simulink model "modelo_planta_EXPERIMENTAL_prueba"  (R2025b)
settings: Solver=FixedStepAuto  StartTime=0.0  StopTime=inf  FixedStep=Ts2  MaxStep=1e-3  RelTol=1e-3
undefined symbols (not defined in the file): ah_max, at_max, bcx, bcy, bh_eq, bhb, bhEb, bhwu, bt, bt_eq, btb, btw, counter_limit, DiscIntNeverNeededParam, g, h_vec_inicial, Hc, ih, is_scanned_vec_inicial, it, Jh_eq, Jt_eq, Kcy, khwu, Ki_h, Ki_t, Kp_h, Kp_t, Ktw, lambda, Lh, Lh0, lh_0, Lt, magnitude, Mc_max, Ms, Mt, N_xt, P_nom, periodo_pulsos, rhd, rtd, tau_hm, tau_tm, Thb_Max, ThEb_Max, Thm_0, Thm_Max, titahm_0, titatm_0, Ts0, Ts1, Ts2, Ttb_Max, Ttm_0, Ttm_Max, vh_0, vh_max_unloaded, vh_nom ... (+20)
libraries: simulink x17, simulink_extras x2, sl3dlib x1, dspnetwork x1
(part 1 of 2)
settings Model: PacingRate=5  Creator=Nahuel  LastModifiedBy=rodri
settings SolverCC: ZeroCrossControl=DisableAll
settings DebuggingCC: UnderSpecifiedDimensionMsg=warning
settings SFSimCC: SimTargetLang=C++  SimDLTargetLibrary=mkl-dnn
settings RTWCC: GPUComputeCapability=3.5
settings ConfigComp: PLC_TargetIDE=codesys35  PLC_MultiTBSigbuilderTimeRange=off  PLC_FoldFBCallOutputVar=off  PLC_RemoveUnusedSSMethodCallArguments=off  PLC_UseCallOutputArgSyntax=off  PLC_EnableUnsignedAndDoubleTypes=off  PLC_EnableUDTSplitting=off  PLC_MaxFieldsInUDT=500.0  PLC_InlineEnumCastFunction=off  PLC_RTWMaxIdLength=31.0  PLC_RollThreshold=5.0  PLC_ActiveTab=0.0  PLC_EnableStringLiteralTB=on  PLC_Enable64bitIntSupport=off

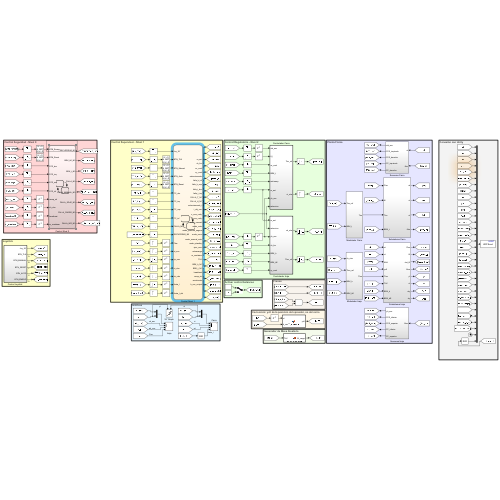
[thumbnail: Simulink's stored preview of the top-level diagram]
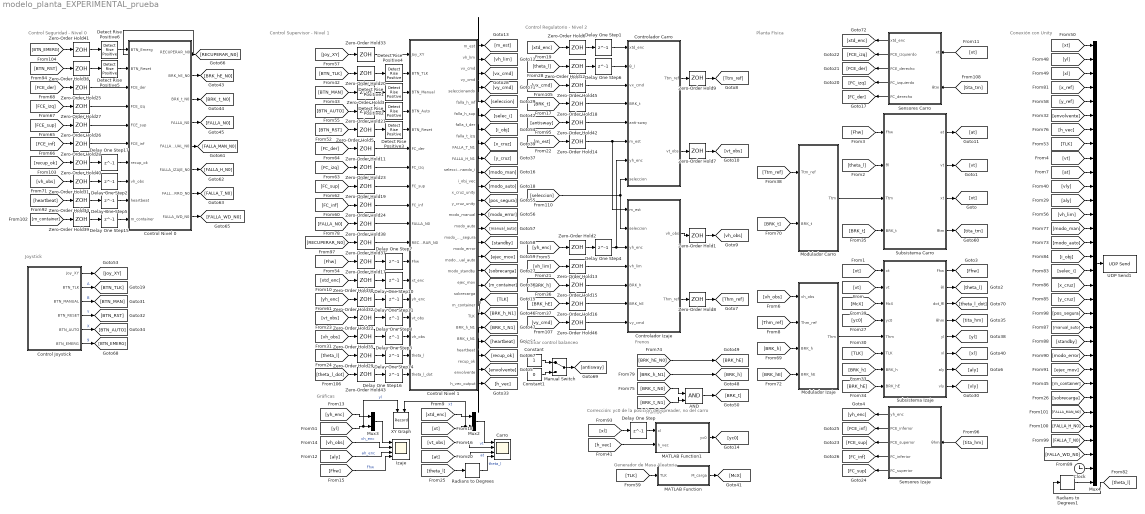
== system modelo_planta_EXPERIMENTAL_prueba ==
  note: Activar control balanceo
  note: Generador de Masa Aleatoria
  note: Frenos
  note: Corrección: yc0 de la posición del spreader, no del carro
  note: Joystick
  note: Control Seguridad - Nivel 0
  note: Control Regulatorio - Nivel 2
  note: Control Supervisor - Nivel 1
  note: Conexión con Unity
  note: Planta Física
  note: Gráficas
  AND : Logic  IconShape=distinctive  AllPortsSameDT=off  OutDataTypeStr=boolean
  Carro : Scope  NumInputPorts=4
      settings: AxesScalingNumUpdates=5  ActiveDisplayYMinimum=-26.90845  ActiveDisplayYMaximum=42.17601
  Clock : Clock
  Constant : Constant
  Constant1 : Constant  Value=0
  "Control Joystick " : Subsystem  TreatAsAtomicUnit=on  SystemSampleTime=Ts2
  Control Nivel 0 : Stateflow chart  Priority=1  TreatAsAtomicUnit=on  SystemSampleTime=Ts0
      settings: PortSchema="{\"entries\":[{\"content\":{\"sides\":[{\"content\":{\"connectorIds\":[\"In1\",\"In7\",\"In2\",\"In5\",\"In3\",\"In6\",\"In10\",\"In4\",\"In8\",\"In9\"]},\"type\":\"ConnectorPlacement.EquallySpacedRectSide\",\"uuid\":\"72248b79-25cb-4c81-9f00-8922a9a1cf34\"},{\"content\":{\"connectorIds\":[\"Out4\",\"Out2\",\"Out3\",\"Out1\",\"Out5\",\"Out6\",\"Out7\",\"Out8\"],\"side\":\"RIGHT\"},\"type\":\"ConnectorPlacement.EquallySpacedRectSide\",\"uuid\":\"f4bfcd12-c204-46a9-9a4b-20ccb9bfcfbb\"},{\"content\":{\"side\":\"TOP\"},\"type\":\"ConnectorPlacement.EquallySpacedRectSide\",\"uuid\":\"f84291a0-0f0e-4f0d-b220-c2febce5b448\"}]},\"type\":\"ConnectorPlacement.EquallySpacedConnector\",\"uuid\":\"3b165743-ae9e-4544-8961-e71410288a4b\"}],\"packageUris\":[\"http://schema.mathworks.com/mf0/Connector/R2020b\"],\"version\":\"1.0\"}"
  Control Nivel 1 : Stateflow chart  Priority=2  TreatAsAtomicUnit=on  SystemSampleTime=Ts1
      settings: PortSchema="{\"entries\":[{\"content\":{\"sides\":[{\"content\":{\"connectorIds\":[\"In5\",\"In4\",\"In6\",\"In7\",\"In8\",\"In9\",\"In11\",\"In10\",\"In12\",\"In15\",\"In16\",\"In3\",\"In18\",\"In13\",\"In2\",\"In14\",\"In17\",\"In1\"]},\"type\":\"ConnectorPlacement.EquallySpacedRectSide\",\"uuid\":\"72765c9f-68bf-44f3-92f3-3edecb9ca866\"},{\"content\":{\"connectorIds\":[\"Out1\",\"Out2\",\"Out22\",\"Out24\",\"Out25\",\"Out26\",\"Out27\",\"Out28\",\"Out29\",\"Out30\",\"Out31\",\"Out9\",\"Out10\",\"Out11\",\"Out12\",\"Out7\",\"Out8\",\"Out13\",\"Out14\",\"Out15\",\"Out16\",\"Out17\",\"Out18\",\"Out19\",\"Out5\",\"Out3\",\"Out4\",\"Out20\",\"Out21\",\"Out23\",\"Out6\"],\"side\":\"RIGHT\"},\"type\":\"ConnectorPlacement.EquallySpacedRectSide\",\"uuid\":\"a6939ff5-eef8-44e2-80ea-5356e254e9e8\"},{\"content\":{\"side\":\"TOP\"},\"type\":\"ConnectorPlacement.EquallySpacedRectSide\",\"uuid\":\"0bd5f797-ecd4-419a-b4ec-9e10260d270a\"},{\"content\":{\"side\":\"BOTTOM\"},\"type\":\"ConnectorPlacement.EquallySpacedRectSide\",\"uuid\":\"7945275f-dab8-4c32-b5c3-f64b82fddda0\"}]},\"type\":\"ConnectorPlacement.EquallySpacedConnector\",\"uuid\":\"3d3cbadb-c70b-461a-afd4-e8d4b160ddcd\"}],\"packageUris\":[\"http://schema.mathworks.com/mf0/Connector/R2020b\"],\"version\":\"1.0\"}"
  Controlador Carro : Subsystem  Priority=3  TreatAsAtomicUnit=on  SystemSampleTime=Ts2
  Controlador Izaje : Subsystem  Priority=3  TreatAsAtomicUnit=on  SystemSampleTime=Ts2
  Delay One Step : Delay  DelayLength=1  InitialCondition=xl_0
  Delay One Step1 : Delay  DelayLength=1  InitialCondition=xtd_0
  Delay One Step10 : Delay  DelayLength=1  InitialCondition=xt_0
  Delay One Step11 : Delay  DelayLength=1  InitialCondition=yh_0
  Delay One Step{2..3,5..6,8,14..17} (9 alike) : Delay  DelayLength=1  InitialCondition=0
  Delay One Step4 : Delay  DelayLength=1  InitialCondition=yh_0
  Delay One Step7 : Delay  DelayLength=1
  Detect Rise Positive{1..6} (6 alike) : simulink/Logic and Bit Operations/Detect Rise Positive  vinit=0  OutDataTypeStr=boolean
  Izaje : Scope  NumInputPorts=4
      settings: ActiveDisplayYMinimum=-22.31965  ActiveDisplayYMaximum=45.47272
  MATLAB Function : MATLAB Function  TreatAsAtomicUnit=on
  MATLAB Function1 : MATLAB Function  TreatAsAtomicUnit=on
  Manual Switch : ManualSwitch
  Modulador Carro : Subsystem
  Modulador Izaje : Subsystem
  Mux2 : Mux  Inputs=2
  Mux3 : Mux  Inputs=2
  Mux4 : Mux  Inputs=32
  Radians to Degrees : simulink_extras/Transformations/Radians to Degrees
  Radians to Degrees1 : simulink_extras/Transformations/Radians to Degrees
  Sensores Carro : Subsystem
  Sensores Izaje : Subsystem
  Subsistema Carro : Subsystem
  Subsistema Izaje : Subsystem
  UDP Send1 : dspnetwork/UDP Send  remoteURL='127.0.0.1'  remotePort=1234  localURL='0.0.0.0'  localPortSource=Automatically determine  localPort=-1  sendBufferSize=8192  sampletime=-1  blockPlatform=HOST  separateLengthPort=0
  XY Graph : Record  NumPorts=2.0  FileSettingsInternal="{\"entries\":[{\"content\":{\"excelSettings\":{\"content\":{},\"type\":\"Streamout.ExcelSettings\"},\"parquetSettings\":{\"content\":{},\"type\":\"Streamout.ParquetSettings\"}},\"type\":\"Streamout.FileSettingStorage\",\"uuid\":\"\"}],\"packageUris\":[\"http:\\/\\/schema.mathworks.com\\/mf0\\/streamout_blocks\\/R2020a\"],\"version\":\"1.0\"}"  FrameSettings=[0, 0]  Layout=[1 1]  SignalsInternal="{\"entries\":[{\"content\":{\"signals\":[{\"content\":{\"blockPath\":[],\"dimensions\":[1],\"domain\":\"\",\"lineColor\":\"#a2142f\",\"plots\":[ 1 ],\"port\":1,\"sid\":[\"\"],\"signalID\":1,\"signalName\":\"yl\"},\"type\":\"RecordBlkView.Signal\",\"uuid\":\"\"},{\"content\":{\"blockPath\":[],\"dimensions\":[1],\"domain\":\"\",\"lineColor\":\"#139fff\",\"plots\":[ 1 ],\"port\":2,\"sid\":[\"\"],\"signalID\":2,\"signalName\":\"xt\"},\"type\":\"RecordBlkView.Signal\",\"uuid\":\"\"}]},\"type\":\"RecordBlkView.InputSignals\",\"uuid\":\"\"}],\"packageUris\":[\"http:\\/\\/schema.mathworks.com\\/mf0\\/streamout_blocks\\/R2020a\"],\"version\":\"1.0\"}"  VisualizationBindings="{\"xyplotplugin\":{\"info\":[{\"series\":[{\"bindingParametersList\":[{\"parameter\":\"X-Axis\",\"signalID\":2,\"signalName\":\"xt\"},{\"parameter\":\"Y-Axis\",\"signalID\":1,\"signalName\":\"yl\"}],\"seriesID\":0}],\"subplotID\":1}]}}"  CompatibilityTag=XY
  Zero-Order Hold{1..2,6..9,12..16,18,42,45..46} (15 alike) : ZeroOrderHold  SampleTime=Ts2
  Zero-Order Hold{3,5,11,17,19..24,29..30,32..33,35,37..38,43} (18 alike) : ZeroOrderHold  SampleTime=Ts1
  Zero-Order Hold{25..28,31,34,36,39..41} (10 alike) : ZeroOrderHold  SampleTime=Ts0
  wires:
  [Thm_ref] -> Modulador Izaje/2(Thm_ref)
  [vh_obs] -> Izaje/2  "vh_enc"
  Sensores Izaje/4(FC_inferior) -> [FC_inf]
  Delay One Step4/1 -> Controlador Carro/7(yh_enc), Controlador Izaje/3(yh_enc)
  Sensores Izaje/1(yh_enc) -> [yh_enc]
  [BRK_hE] -> Subsistema Izaje/8(BRK_hE)
  Subsistema Izaje/1(Fhw) -> [Fhw]
  Controlador Izaje/2(Thm_ref) -> Zero-Order Hold8/1
  [xt] -> Sensores Carro/1(xt)
  [BRK_h] -> Subsistema Izaje/7(BRK_h)
  Sensores Carro/4(FC_izquierdo) -> [FC_izq]
  [m_est] -> Zero-Order Hold14/1
  Zero-Order Hold2/1 -> Delay One Step4/1
  Zero-Order Hold6/1 -> Delay One Step1/1
  Subsistema Carro/1(at) -> [at]
  [theta_l] -> Subsistema Carro/2(θl)
  [vt] -> Subsistema Izaje/2(vt)
  [xt] -> Subsistema Izaje/1(xt)
  Delay One Step1/1 -> Controlador Carro/1(xtd_enc)
  [aly] -> Izaje/3  "ah_enc"
  Zero-Order Hold8/1 -> [Thm_ref]
  [vh_lim] -> Zero-Order Hold13/1
  Subsistema Carro/3(xt) -> [xt]
  [Fhw] -> Subsistema Carro/1(Fhw)
  Sensores Carro/2(FCE_izquierdo) -> [FCE_izq]
  [yh_enc] -> Zero-Order Hold2/1
  [xtd_enc] -> Zero-Order Hold6/1
  Zero-Order Hold9/1 -> [Ttm_ref]
  Controlador Carro/1(Ttm_ref) -> Zero-Order Hold9/1
  [TLK] -> Subsistema Izaje/6(TLK)
  Sensores Izaje/2(FCE_inferior) -> [FCE_inf]
  Sensores Izaje/3(FCE_superior) -> [FCE_sup]
  Sensores Izaje/5(FC_superior) -> [FC_sup]
  Sensores Carro/3(FCE_derecho) -> [FCE_der]
  Subsistema Izaje/2(θl) -> [theta_l]
  [McX] -> Subsistema Izaje/3(McX)
  Subsistema Carro/2(vt) -> [vt]
  Sensores Carro/5(FC_derecho) -> [FC_der]
  [BRK_t] -> Subsistema Carro/4(BRK_t)
  [BRK_h] -> Zero-Order Hold15/1
  [BRK_hE] -> Zero-Order Hold16/1
  [Ttm_ref] -> Modulador Carro/1(Ttm_ref)
  [BRK_t] -> Zero-Order Hold18/1
  [yh_enc] -> Mux3/1
  [vh_obs] -> Modulador Izaje/1(vh_obs)
  Delay One Step6/1 -> Controlador Carro/2(θ_l)
  [theta_l] -> Zero-Order Hold12/1
  Zero-Order Hold12/1 -> Delay One Step6/1
  Modulador Izaje/1(Thm) -> Subsistema Izaje/5(Thm)
  Modulador Carro/1(Ttm) -> Subsistema Carro/3(Ttm)
  Mux3/1 -> Izaje/1
  Subsistema Izaje/5(yl) -> [yl]
  Subsistema Izaje/6(xl) -> [xl]
  [Fhw] -> Izaje/4  "Fhw"
  Subsistema Izaje/7(aly) -> [aly]
  [yl] -> Mux3/2, XY Graph/1  "yl"
  Control Nivel 1/1(m_est) -> [m_est]
  Control Nivel 1/2(vh_lim) -> [vh_lim]
  Zero-Order Hold13/1 -> Controlador Izaje/4(vh_lim)
  Zero-Order Hold14/1 -> Controlador Izaje/1(m_est), Controlador Carro/6(m_est)
  Zero-Order Hold15/1 -> Controlador Izaje/5(BRK_h)
  Zero-Order Hold16/1 -> Controlador Izaje/6(BRK_hE)
  Zero-Order Hold17/1 -> Delay One Step7/1
  Delay One Step7/1 -> Control Nivel 1/3(Fhw)
  [Fhw] -> Zero-Order Hold17/1
  Zero-Order Hold18/1 -> Controlador Carro/4(BRK_t)
  [BTN_TLK] -> Zero-Order Hold20/1
  Zero-Order Hold20/1 -> Detect Rise Positive4/1
  Zero-Order Hold11/1 -> Control Nivel 1/9(FC_der)
  Zero-Order Hold19/1 -> Control Nivel 1/10(FC_sup)
  Zero-Order Hold23/1 -> Control Nivel 1/11(FC_izq)
  Zero-Order Hold24/1 -> Control Nivel 1/12(FC_inf)
  [FC_izq] -> Zero-Order Hold23/1
  [FC_der] -> Zero-Order Hold11/1
  [FC_sup] -> Zero-Order Hold19/1
  [FC_inf] -> Zero-Order Hold24/1
  Zero-Order Hold25/1 -> Control Nivel 0/2(FCE_der)
  Zero-Order Hold26/1 -> Control Nivel 0/3(FCE_sup)
  Zero-Order Hold27/1 -> Control Nivel 0/5(FCE_izq)
  Zero-Order Hold28/1 -> Control Nivel 0/6(FCE_inf)
  [FCE_der] -> Zero-Order Hold25/1
  [FCE_izq] -> Zero-Order Hold27/1
  [FCE_sup] -> Zero-Order Hold26/1
  [FCE_inf] -> Zero-Order Hold28/1
  [BRK_h] -> Modulador Izaje/3(BRK_h)
  [vh_obs] -> Zero-Order Hold31/1
  Zero-Order Hold31/1 -> Delay One Step2/1
  [BRK_hE] -> Modulador Izaje/4(BRK_hE)
  [BRK_t] -> Modulador Carro/2(BRK_t)
  Control Nivel 0/2(BRK_hE_N0) -> [BRK_hE_N0]
  Control Nivel 0/3(BRK_t_N0) -> [BRK_t_N0]
  [xtd_enc] -> Zero-Order Hold30/1
  [yh_enc] -> Zero-Order Hold32/1
  Zero-Order Hold30/1 -> Delay One Step10/1
  Zero-Order Hold32/1 -> Delay One Step11/1
  Delay One Step11/1 -> Control Nivel 1/13(yh_enc)
  Control Nivel 0/1(FALLA_N0) -> [FALLA_N0]
  [FALLA_N0] -> Zero-Order Hold38/1
  Control Nivel 1/3(BRK_h_N1) -> [BRK_h_N1]
  Control Nivel 1/4(BRK_t_N1) -> [BRK_t_N1]
  [BRK_t_N0] -> AND/1
  [BRK_t_N1] -> AND/2
  [BRK_h_N1] -> [BRK_h]
  [BRK_hE_N0] -> [BRK_hE]
  AND/1 -> [BRK_t]
  [BTN_MAN] -> Zero-Order Hold3/1
  Zero-Order Hold38/1 -> Control Nivel 1/15(FALLA_N0)
  "Control Joystick "/2(BTN_TLK) -> [BTN_TLK]  "A"
  "Control Joystick "/1(Joy_XY) -> [Joy_XY]
  [Joy_XY] -> Zero-Order Hold33/1
  Zero-Order Hold33/1 -> Control Nivel 1/5(Joy_XY)
  Control Nivel 1/5(TLK) -> [TLK]
  Delay One Step16/1 -> Control Nivel 1/1(theta_l_dot)
  Control Nivel 1/6(h_vec_output) -> [h_vec]
  Subsistema Izaje/8(vly) -> [vly]
  "Control Joystick "/5(BTN_AUTO) -> [BTN_AUTO]  "X"
  "Control Joystick "/4(BTN_RESET) -> [BTN_RST]  "Y"
  "Control Joystick "/3(BTN_MANUAL) -> [BTN_MAN]  "B"
  Zero-Order Hold3/1 -> Detect Rise Positive1/1
  [BTN_AUTO] -> Zero-Order Hold21/1
  Zero-Order Hold21/1 -> Detect Rise Positive2/1
  [BTN_RST] -> Zero-Order Hold5/1
  Zero-Order Hold5/1 -> Detect Rise Positive3/1
  [TLK] -> MATLAB Function/1(TLK)
  MATLAB Function/1(M_carga) -> [McX]
  [vh_lim] -> Mux4/13
  [at] -> Mux4/10
  [vt] -> Mux4/9
  [xt] -> Mux4/1
  [envolvente] -> Mux4/6
  [vly] -> Mux4/11
  [h_vec] -> Mux4/7
  [yl] -> Mux4/2
  [y_ref] -> Mux4/5
  [TLK] -> Mux4/8
  [xl] -> Mux4/3
  [x_ref] -> Mux4/4
  Mux4/1 -> UDP Send1/1
  [vt_obs] -> Zero-Order Hold22/1
  Zero-Order Hold22/1 -> Delay One Step8/1
  Delay One Step8/1 -> Control Nivel 1/2(vt_obs)
  [theta_l] -> Zero-Order Hold29/1
  Zero-Order Hold29/1 -> Delay One Step14/1
  Delay One Step14/1 -> Control Nivel 1/17(theta_l)
  Control Nivel 1/7(modo_manual) -> [modo_man]
  Control Nivel 1/8(modo_auto) -> [modo_auto]
  [modo_man] -> Mux4/14
  [modo_auto] -> Mux4/15
  Control Nivel 1/12(y_cruz_unity) -> [y_cruz]
  Control Nivel 1/11(x_cruz_unity) -> [x_cruz]
  Control Nivel 1/9(seleccionando_i) -> [selec_i]
  Control Nivel 1/10(i_obj_vec) -> [i_obj]
  [i_obj] -> Mux4/16
  [selec_i] -> Mux4/17
  [x_cruz] -> Mux4/18
  [y_cruz] -> Mux4/19
  Control Nivel 1/13(modo_posicion_segura) -> [pos_segura]
  Control Nivel 1/14(modo_error) -> [modo_error]
  Control Nivel 1/15(modo_manual_auto) -> [manual_auto]
  Control Nivel 1/16(modo_standby) -> [standby]
  [pos_segura] -> Mux4/20
  [manual_auto] -> Mux4/21
  [standby] -> Mux4/22
  [modo_error] -> Mux4/23
  Control Nivel 1/17(ejec_mov) -> [ejec_mov]
  [ejec_mov] -> Mux4/24
  Control Nivel 1/19(m_container) -> [m_container]
  Control Nivel 1/18(sobrecarga) -> [sobrecarga]
  [m_container] -> Mux4/25
  [sobrecarga] -> Mux4/26
  MATLAB Function1/1(yc0) -> [yc0]
  [xl] -> Delay One Step/1
  Delay One Step/1 -> MATLAB Function1/1(xl)
  [h_vec] -> MATLAB Function1/2(h_vec)
  [yc0] -> Subsistema Izaje/4(yc0)
  [BTN_RST] -> Zero-Order Hold36/1
  [aly] -> Mux4/12
  Control Nivel 0/5(FALLA_MANUAL_N0) -> [FALLA_MAN_N0]
  Control Nivel 0/6(FALLA_IZAJE_N0) -> [FALLA_H_N0]
  Control Nivel 0/7(FALLA_CARRO_N0) -> [FALLA_T_N0]
  Control Nivel 1/20(heartbeat) -> [heartbeat]
  [heartbeat] -> Zero-Order Hold34/1
  Zero-Order Hold34/1 -> Delay One Step5/1
  Zero-Order Hold36/1 -> Detect Rise Positive5/1
  Delay One Step5/1 -> Control Nivel 0/8(heartbeat)
  Control Nivel 0/8(FALLA_WD_N0) -> [FALLA_WD_N0]
  [FALLA_MAN_N0] -> Mux4/27
  [FALLA_H_N0] -> Mux4/28
  [FALLA_T_N0] -> Mux4/29
  [FALLA_WD_N0] -> Mux4/30
  Control Nivel 0/4(RECUPERAR_N0) -> [RECUPERAR_N0]
  [RECUPERAR_N0] -> Zero-Order Hold37/1
  Zero-Order Hold37/1 -> Control Nivel 1/16(RECUPERAR_N0)
  [m_container] -> Zero-Order Hold39/1
  Zero-Order Hold39/1 -> Delay One Step15/1
  Delay One Step15/1 -> Control Nivel 0/9(m_container)
  Control Nivel 1/21(recup_ok) -> [recup_ok]
  [recup_ok] -> Zero-Order Hold40/1
  Zero-Order Hold40/1 -> Delay One Step17/1
  "Control Joystick "/6(BTN_EMERG) -> [BTN_EMERG]  "9"
  Zero-Order Hold41/1 -> Detect Rise Positive6/1
  [BTN_EMERG] -> Zero-Order Hold41/1
  Detect Rise Positive1/1 -> Control Nivel 1/6(BTN_Manual)
  Detect Rise Positive2/1 -> Control Nivel 1/7(BTN_Auto)
  Detect Rise Positive3/1 -> Control Nivel 1/8(BTN_Reset)
  Detect Rise Positive4/1 -> Control Nivel 1/4(BTN_TLK)
  Detect Rise Positive5/1 -> Control Nivel 0/7(BTN_Reset)
  Detect Rise Positive6/1 -> Control Nivel 0/1(BTN_Emerg)
  Zero-Order Hold42/1 -> Controlador Carro/5(anti-sway)
  [antisway] -> Zero-Order Hold42/1
  Mux2/1 -> Carro/1
  [theta_l] -> Radians to Degrees/1
  [xt] -> Mux2/2, XY Graph/2  "xt"
  [vt_obs] -> Carro/2  "vt"
  Radians to Degrees/1 -> Carro/4  "theta_l"
  [at] -> Carro/3  "at"
  [xtd_enc] -> Mux2/1
  [theta_l_dot] -> Zero-Order Hold43/1
  Zero-Order Hold43/1 -> Delay One Step16/1
  Subsistema Izaje/3(dot_θl) -> [theta_l_dot]
  Control Nivel 1/22(vx_cmd) -> [vx_cmd]
  Control Nivel 1/24(vy_cmd) -> [vy_cmd]
  [vx_cmd] -> Zero-Order Hold45/1
  Zero-Order Hold45/1 -> Controlador Carro/3(vx_cmd)
  [vy_cmd] -> Zero-Order Hold46/1
  Zero-Order Hold46/1 -> Controlador Izaje/7(vy_cmd)
  Controlador Carro/2(vt_obs) -> Zero-Order Hold7/1
  Zero-Order Hold7/1 -> [vt_obs]
  Delay One Step10/1 -> Control Nivel 1/18(xt_enc)
  Sensores Carro/1(xtd_enc) -> [xtd_enc]
  Controlador Izaje/1(vh_obs) -> Zero-Order Hold1/1
  Zero-Order Hold1/1 -> [vh_obs]
  Delay One Step2/1 -> Control Nivel 0/4(vh_obs)
  Constant/1 -> Manual Switch/1
  Manual Switch/1 -> [antisway]
  Constant1/1 -> Manual Switch/2
  [vh_obs] -> Zero-Order Hold35/1
  Zero-Order Hold35/1 -> Delay One Step3/1
  Delay One Step3/1 -> Control Nivel 1/14(vh_obs)
  Control Nivel 1/23(envolvente) -> [envolvente]
  Delay One Step17/1 -> Control Nivel 0/10(recup_ok)
  Subsistema Izaje/4(θhm) -> [tita_hm]
  [tita_hm] -> Sensores Izaje/1(θhm)
  Subsistema Carro/4(θtm) -> [tita_tm]
  [tita_tm] -> Sensores Carro/2(θtm)
  Clock/1 -> Mux4/31
  [theta_l] -> Radians to Degrees1/1
  Radians to Degrees1/1 -> Mux4/32
  Control Nivel 1/25(seleccionando) -> [seleccion]
  [seleccion] -> Controlador Izaje/2(seleccion), Controlador Carro/8(seleccion)

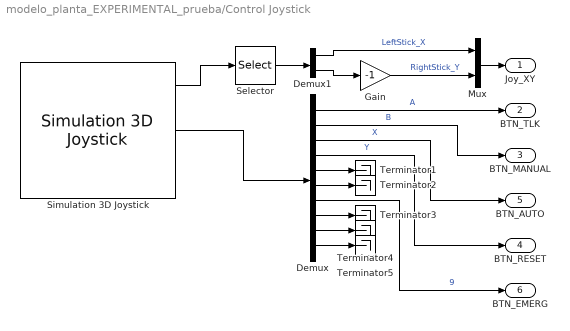
== system modelo_planta_EXPERIMENTAL_prueba/Control Joystick  ==
  Demux : Demux  Outputs=10
  Demux1 : Demux  Outputs=2
  Gain : Gain  Gain=-1
  Mux : Mux  Inputs=2
  Selector : Selector  InputPortWidth=5  IndexOptions=Index vector (dialog)  Indices=[1 5]  OutputSizes=1
  Simulation 3D Joystick : sl3dlib/Simulation 3D/Hardware Interface/Simulation 3D Joystick  joyid=1  adjustports=on  forcefeed=off
  Terminator{1..5} (5 alike) : Terminator
  Joy_XY : Outport
  BTN_TLK : Outport  Port=2
  BTN_MANUAL : Outport  Port=3
  BTN_RESET : Outport  Port=4
  BTN_AUTO : Outport  Port=5
  BTN_EMERG : Outport  Port=6
  wires:
  Demux/1 -> BTN_TLK/1  "A"
  Demux1/2 -> Gain/1
  Demux1/1 -> Mux/1  "LeftStick_X"
  Selector/1 -> Demux1/1
  Simulation 3D Joystick/1 -> Selector/1
  Gain/1 -> Mux/2  "RightStick_Y"
  Simulation 3D Joystick/2 -> Demux/1
  Demux/2 -> BTN_MANUAL/1  "B"
  Demux/3 -> BTN_AUTO/1  "X"
  Demux/4 -> BTN_RESET/1  "Y"
  Mux/1 -> Joy_XY/1
  Demux/5 -> Terminator1/1
  Demux/6 -> Terminator2/1
  Demux/8 -> Terminator3/1
  Demux/9 -> Terminator4/1
  Demux/10 -> Terminator5/1
  Demux/7 -> BTN_EMERG/1  "9"

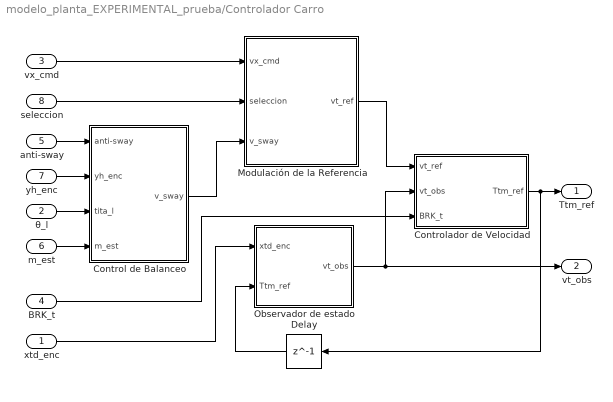
== system modelo_planta_EXPERIMENTAL_prueba/Controlador Carro ==
  xtd_enc : Inport
  θ_l : Inport  Port=2
  vx_cmd : Inport  Port=3
  BRK_t : Inport  Port=4
  anti-sway : Inport  Port=5
  m_est : Inport  Port=6
  yh_enc : Inport  Port=7
  seleccion : Inport  Port=8
  Control de Balanceo : Subsystem
  Controlador de Velocidad : Subsystem
  Delay : Delay  DelayLength=1  InitialCondition=Ttm_0
  Modulación de la Referencia : Subsystem
  Observador de estado : Subsystem  TreatAsAtomicUnit=on  SystemSampleTime=Ts2
  Ttm_ref : Outport
  vt_obs : Outport  Port=2
  wires:
  Modulación de la Referencia/1(vt_ref) -> Controlador de Velocidad/1(vt_ref)
  Controlador de Velocidad/1(Ttm_ref) -> Ttm_ref/1, Delay/1
  xtd_enc/1 -> Observador de estado/1(xtd_enc)
  Delay/1 -> Observador de estado/2(Ttm_ref)
  Control de Balanceo/1(v_sway) -> Modulación de la Referencia/3(v_sway)
  yh_enc/1 -> Control de Balanceo/2(yh_enc)
  θ_l/1 -> Control de Balanceo/3(tita_l)
  m_est/1 -> Control de Balanceo/4(m_est)
  BRK_t/1 -> Controlador de Velocidad/3(BRK_t)
  vx_cmd/1 -> Modulación de la Referencia/1(vx_cmd)
  anti-sway/1 -> Control de Balanceo/1(anti-sway)
  Observador de estado/1(vt_obs) -> Controlador de Velocidad/2(vt_obs), vt_obs/1
  seleccion/1 -> Modulación de la Referencia/2(seleccion)

== system modelo_planta_EXPERIMENTAL_prueba/Controlador Izaje ==
  m_est : Inport
  seleccion : Inport  Port=2
  yh_enc : Inport  Port=3
  vh_lim : Inport  Port=4
  BRK_h : Inport  Port=5
  BRK_hE : Inport  Port=6
  vy_cmd : Inport  Port=7
  AND : Logic  IconShape=distinctive  AllPortsSameDT=off  OutDataTypeStr=boolean
  Controlador de Velocidad : Subsystem  TreatAsAtomicUnit=on  SystemSampleTime=Ts2
  Delay One Step : Delay  DelayLength=1  InitialCondition=Thm_0
  Modulación de la Referencia : Subsystem  TreatAsAtomicUnit=on  SystemSampleTime=Ts2
  Observador de estado : Subsystem  TreatAsAtomicUnit=on  SystemSampleTime=Ts2
  vh_obs : Outport
  Thm_ref : Outport  Port=2
  wires:
  yh_enc/1 -> Observador de estado/1(yh_enc)
  Observador de estado/1(vh_obs) -> Controlador de Velocidad/3(vh_obs), vh_obs/1
  Modulación de la Referencia/1(vh_ref) -> Controlador de Velocidad/2(vh_ref)
  vh_lim/1 -> Modulación de la Referencia/1(vh_lim)
  AND/1 -> Controlador de Velocidad/4(BRK)
  Controlador de Velocidad/1(Thm_ref) -> Delay One Step/1, Thm_ref/1
  Delay One Step/1 -> Observador de estado/2(Thm_ref)
  m_est/1 -> Controlador de Velocidad/1(m_est)
  BRK_h/1 -> AND/1
  BRK_hE/1 -> AND/2
  vy_cmd/1 -> Modulación de la Referencia/3(vy_cmd)
  seleccion/1 -> Modulación de la Referencia/2(seleccion)

== system modelo_planta_EXPERIMENTAL_prueba/Modulador Carro ==
  Ttm_ref : Inport
  BRK_t : Inport  Port=2
  Constant1 : Constant  Value=0
  Gain2 : Gain  Gain=1/tau_tm
  Integrator : Integrator  InitialCondition=Ttm_0
  Saturation : Saturate  UpperLimit=Ttm_Max  LowerLimit=-Ttm_Max
  Sum : Sum  Inputs=|+-
  Switch : Switch  Criteria=u2 > Threshold  SaturateOnIntegerOverflow=off  InputSameDT=off
  Ttm : Outport
  wires:
  Saturation/1 -> Sum/1  "Ttm_lim"
  Sum/1 -> Gain2/1
  Gain2/1 -> Integrator/1
  Integrator/1 -> Ttm/1, Sum/2
  Ttm_ref/1 -> Switch/1
  BRK_t/1 -> Switch/2
  Switch/1 -> Saturation/1
  Constant1/1 -> Switch/3

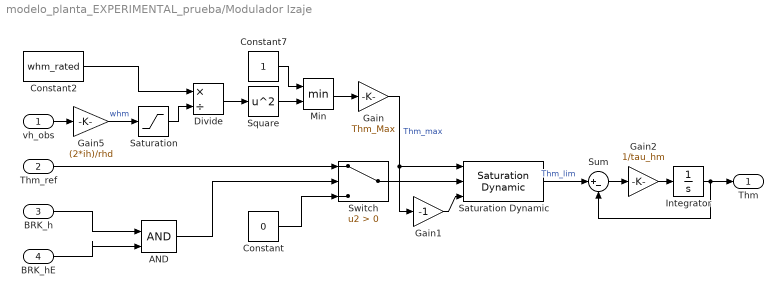
== system modelo_planta_EXPERIMENTAL_prueba/Modulador Izaje ==
  vh_obs : Inport
  Thm_ref : Inport  Port=2
  BRK_h : Inport  Port=3
  BRK_hE : Inport  Port=4
  AND : Logic  IconShape=distinctive  AllPortsSameDT=off  OutDataTypeStr=boolean
  Constant : Constant  Value=0
  Constant2 : Constant  Value=whm_rated
  Constant7 : Constant
  Divide : Product  Inputs=*/
  Gain : Gain  Gain=Thm_Max
  Gain1 : Gain  Gain=-1
  Gain2 : Gain  Gain=1/tau_hm
  Gain5 : Gain  Gain=(2*ih)/rhd
  Integrator : Integrator  InitialCondition=Thm_0
  Min : MinMax  Inputs=2
  Saturation : Saturate  UpperLimit=inf  LowerLimit=whm_rated
  Saturation Dynamic : simulink/Discontinuities/Saturation Dynamic  OutMin=[]  OutMax=[]  OutDataTypeStr=Inherit: Same as second input  OutDataType=fixdt(1, 16)  OutScaling=2^-10  DoSatur=off
  Square : Math  Operator=square
  Sum : Sum  Inputs=|+-
  Switch : Switch  Criteria=u2 > Threshold  SaturateOnIntegerOverflow=off  InputSameDT=off
  Thm : Outport
  wires:
  Constant2/1 -> Divide/1
  Min/1 -> Gain/1
  Constant7/1 -> Min/1
  Gain/1 -> Gain1/1, Saturation Dynamic/1  "Thm_max"
  Saturation/1 -> Divide/2
  Square/1 -> Min/2
  Divide/1 -> Square/1
  vh_obs/1 -> Gain5/1
  Gain1/1 -> Saturation Dynamic/3
  Saturation Dynamic/1 -> Sum/1  "Thm_lim"
  Sum/1 -> Gain2/1
  Gain2/1 -> Integrator/1
  Integrator/1 -> Thm/1, Sum/2
  Thm_ref/1 -> Switch/1
  BRK_h/1 -> AND/1
  Switch/1 -> Saturation Dynamic/2
  BRK_hE/1 -> AND/2
  AND/1 -> Switch/2
  Gain5/1 -> Saturation/1  "whm"
  Constant/1 -> Switch/3

== system modelo_planta_EXPERIMENTAL_prueba/Sensores Carro ==
  xt : Inport
  θtm : Inport  Port=2
  Encoder Carro : Subsystem
  Fines de carrera carro (rieles) : Subsystem
  xtd_enc : Outport
  FCE_izquierdo : Outport  Port=2
  FCE_derecho : Outport  Port=3
  FC_izquierdo : Outport  Port=4
  FC_derecho : Outport  Port=5
  wires:
  Fines de carrera carro (rieles)/1(FC_derecho) -> FC_derecho/1
  θtm/1 -> Encoder Carro/1(θtm)
  Fines de carrera carro (rieles)/2(FC_izquierdo) -> FC_izquierdo/1
  Fines de carrera carro (rieles)/3(FCE_derecho) -> FCE_derecho/1
  Fines de carrera carro (rieles)/4(FCE_izquierdo) -> FCE_izquierdo/1
  xt/1 -> Fines de carrera carro (rieles)/1(xt)
  Encoder Carro/1(xtd_enc) -> xtd_enc/1

== system modelo_planta_EXPERIMENTAL_prueba/Sensores Izaje ==
  θhm : Inport
  Encoder Izaje : Subsystem
  Fines de carrera izaje (tambor) : Subsystem
  yh_enc : Outport
  FCE_inferior : Outport  Port=2
  FCE_superior : Outport  Port=3
  FC_inferior : Outport  Port=4
  FC_superior : Outport  Port=5
  wires:
  Fines de carrera izaje (tambor)/1(FC_superior) -> FC_superior/1
  Fines de carrera izaje (tambor)/4(FCE_inferior) -> FCE_inferior/1
  Fines de carrera izaje (tambor)/2(FC_inferior) -> FC_inferior/1
  Encoder Izaje/1(yh_enc) -> Fines de carrera izaje (tambor)/1(y_enc), yh_enc/1
  θhm/1 -> Encoder Izaje/1(θhm)
  Fines de carrera izaje (tambor)/3(FCE_superior) -> FCE_superior/1

== system modelo_planta_EXPERIMENTAL_prueba/Subsistema Carro ==
  Fhw : Inport
  θl : Inport  Port=2
  Ttm : Inport  Port=3
  BRK_t : Inport  Port=4
  Accionamiento carro : Subsystem
  Dinámica carro : Subsystem
  Fuerza cable carro : Subsystem
  at : Outport
  vt : Outport  Port=2
  xt : Outport  Port=3
  θtm : Outport  Port=4
  wires:
  [Ftw] -> Accionamiento carro/1(Ftw)
  Accionamiento carro/1(θtm) -> θtm/1
  Dinámica carro/1(xt) -> Fuerza cable carro/3(xt), xt/1
  BRK_t/1 -> Accionamiento carro/3(BRK_t)
  [Ftw] -> Dinámica carro/1(Ftw)
  θl/1 -> Dinámica carro/2(θl)
  Ttm/1 -> Accionamiento carro/2(Ttm)
  Fuerza cable carro/1(Ftw) -> [Ftw]
  Dinámica carro/2(vt) -> Fuerza cable carro/4(vt), vt/1
  Accionamiento carro/2(xtd) -> Fuerza cable carro/1(xtd)
  Accionamiento carro/3(vtd) -> Fuerza cable carro/2(vtd)
  Fhw/1 -> Dinámica carro/3(Fhw)
  Dinámica carro/3(at) -> at/1

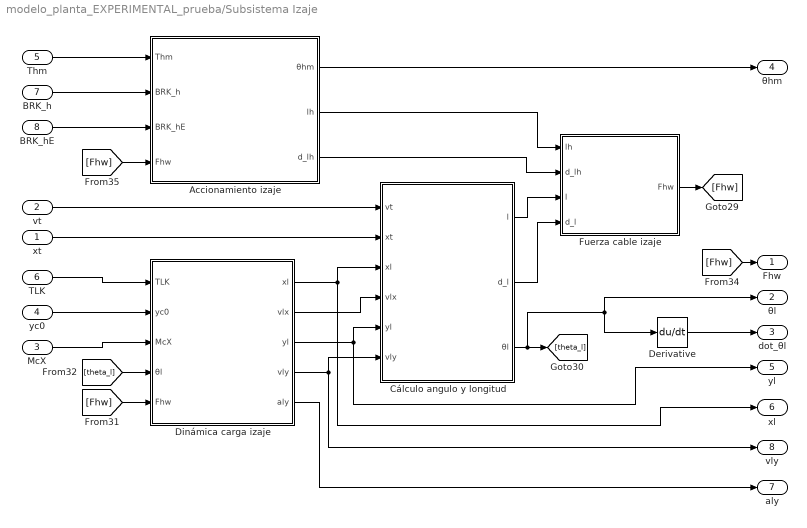
== system modelo_planta_EXPERIMENTAL_prueba/Subsistema Izaje ==
  xt : Inport
  vt : Inport  Port=2
  McX : Inport  Port=3
  yc0 : Inport  Port=4
  Thm : Inport  Port=5
  TLK : Inport  Port=6
  BRK_h : Inport  Port=7
  BRK_hE : Inport  Port=8
  Accionamiento izaje : Subsystem
  Cálculo angulo y longitud : Subsystem
  Derivative : Derivative
  Dinámica carga izaje : Subsystem
  Fuerza cable izaje : Subsystem
  Fhw : Outport
  θl : Outport  Port=2
  dot_θl : Outport  Port=3
  θhm : Outport  Port=4
  yl : Outport  Port=5
  xl : Outport  Port=6
  aly : Outport  Port=7
  vly : Outport  Port=8
  wires:
  vt/1 -> Cálculo angulo y longitud/1(vt)
  Accionamiento izaje/2(lh) -> Fuerza cable izaje/1(lh)
  yc0/1 -> Dinámica carga izaje/2(yc0)
  McX/1 -> Dinámica carga izaje/3(McX)
  Dinámica carga izaje/4(vly) -> vly/1, Cálculo angulo y longitud/6(vly)
  [Fhw] -> Accionamiento izaje/4(Fhw)
  [theta_l] -> Dinámica carga izaje/4(θl)
  xt/1 -> Cálculo angulo y longitud/2(xt)
  BRK_h/1 -> Accionamiento izaje/2(BRK_h)
  Dinámica carga izaje/1(xl) -> Cálculo angulo y longitud/3(xl), xl/1
  Dinámica carga izaje/2(vlx) -> Cálculo angulo y longitud/4(vlx)
  Fuerza cable izaje/1(Fhw) -> [Fhw]
  Cálculo angulo y longitud/1(l) -> Fuerza cable izaje/3(l)
  Accionamiento izaje/1(θhm) -> θhm/1
  Cálculo angulo y longitud/3(θl) -> θl/1, Derivative/1, [theta_l]
  TLK/1 -> Dinámica carga izaje/1(TLK)
  [Fhw] -> Dinámica carga izaje/5(Fhw)
  BRK_hE/1 -> Accionamiento izaje/3(BRK_hE)
  Thm/1 -> Accionamiento izaje/1(Thm)
  Dinámica carga izaje/3(yl) -> Cálculo angulo y longitud/5(yl), yl/1
  Cálculo angulo y longitud/2(d_l) -> Fuerza cable izaje/4(d_l)
  Accionamiento izaje/3(d_lh) -> Fuerza cable izaje/2(d_lh)
  Dinámica carga izaje/5(aly) -> aly/1
  [Fhw] -> Fhw/1
  Derivative/1 -> dot_θl/1

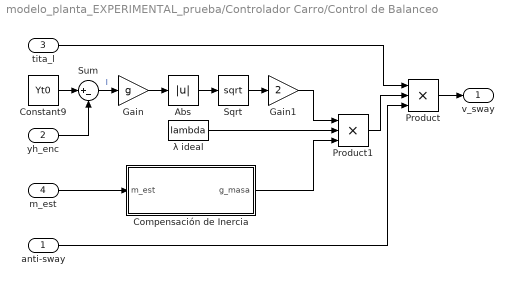
== system modelo_planta_EXPERIMENTAL_prueba/Controlador Carro/Control de Balanceo ==
  anti-sway : Inport
  yh_enc : Inport  Port=2
  tita_l : Inport  Port=3
  m_est : Inport  Port=4
  Abs : Abs  SaturateOnIntegerOverflow=off
  Compensación de Inercia : MATLAB Function  TreatAsAtomicUnit=on
  Constant9 : Constant  Value=Yt0
  Gain : Gain  Gain=g
  Gain1 : Gain  Gain=2
  Product : Product  Inputs=3
  Product1 : Product  Inputs=3
  Sqrt : Sqrt
  Sum : Sum  Inputs=|+-
  λ ideal : Constant  Value=lambda
  v_sway : Outport
  wires:
  Compensación de Inercia/1(g_masa) -> Product1/3
  Gain1/1 -> Product1/1
  Constant9/1 -> Sum/1
  Sqrt/1 -> Gain1/1
  Product/1 -> v_sway/1
  Sum/1 -> Gain/1  "l"
  yh_enc/1 -> Sum/2
  Abs/1 -> Sqrt/1
  λ ideal/1 -> Product1/2
  Gain/1 -> Abs/1
  tita_l/1 -> Product/1
  Product1/1 -> Product/2
  m_est/1 -> Compensación de Inercia/1(m_est)
  anti-sway/1 -> Product/3

== system modelo_planta_EXPERIMENTAL_prueba/Controlador Carro/Controlador de Velocidad ==
  vt_ref : Inport
  vt_obs : Inport  Port=2
  BRK_t : Inport  Port=3
  Discrete-Time Integrator : DiscreteIntegrator  IntegratorMethod=Integration: Trapezoidal  ExternalReset=level  SampleTime=-1  ICPrevOutput=DiscIntNeverNeededParam  ICPrevScaledInput=DiscIntNeverNeededParam
  Gain5 : Gain  Gain=Ki_t
  Gain6 : Gain  Gain=Kp_t
  NOT : Logic  Operator=NOT  IconShape=distinctive  AllPortsSameDT=off  OutDataTypeStr=boolean
  Sum6 : Sum  Inputs=+-
  Sum7 : Sum  Inputs=++|
  Ttm_ref : Outport
  wires:
  Sum6/1 -> Gain6/1, Discrete-Time Integrator/1  "e_v"
  Sum7/1 -> Ttm_ref/1
  Gain5/1 -> Sum7/2
  vt_ref/1 -> Sum6/1
  Gain6/1 -> Sum7/1
  vt_obs/1 -> Sum6/2
  Discrete-Time Integrator/1 -> Gain5/1
  BRK_t/1 -> NOT/1
  NOT/1 -> Discrete-Time Integrator/2

== system modelo_planta_EXPERIMENTAL_prueba/Controlador Carro/Modulación de la Referencia ==
  vx_cmd : Inport
  seleccion : Inport  Port=2
  v_sway : Inport  Port=3
  Constant : Constant  Value=vt_max
  Constant2 : Constant  Value=0
  Gain2 : Gain  Gain=-1
  Rate Limiter : RateLimiter  RisingSlewLimit=at_max  FallingSlewLimit=-at_max  SampleTimeMode=inherited  InitialCondition=vt_0
  Saturation Dynamic : simulink/Discontinuities/Saturation Dynamic  OutMin=[]  OutMax=[]  OutDataTypeStr=Inherit: Same as second input  OutDataType=fixdt(1, 16)  OutScaling=2^-10  DoSatur=off
  Sum1 : Sum  Inputs=++|
  Switch : Switch  Criteria=u2 > Threshold  SaturateOnIntegerOverflow=off  InputSameDT=off
  vt_ref : Outport
  wires:
  v_sway/1 -> Sum1/2
  Saturation Dynamic/1 -> Rate Limiter/1
  Rate Limiter/1 -> vt_ref/1
  Gain2/1 -> Saturation Dynamic/3
  Constant/1 -> Gain2/1, Saturation Dynamic/1
  Sum1/1 -> Saturation Dynamic/2  "vt_cmd"
  Switch/1 -> Sum1/1
  vx_cmd/1 -> Switch/3
  seleccion/1 -> Switch/2
  Constant2/1 -> Switch/1

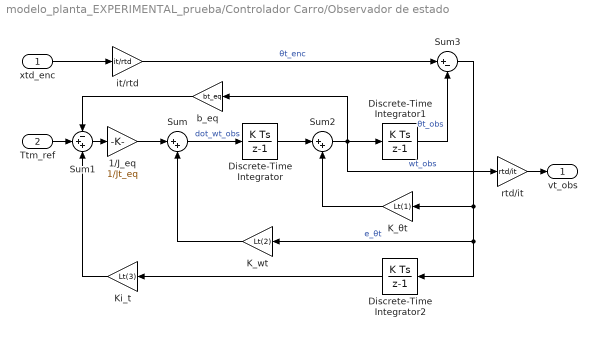
== system modelo_planta_EXPERIMENTAL_prueba/Controlador Carro/Observador de estado ==
  xtd_enc : Inport
  Ttm_ref : Inport  Port=2
  1/J_eq : Gain  Gain=1/Jt_eq
  Discrete-Time Integrator : DiscreteIntegrator  InitialCondition=wtm_0  SampleTime=-1  ICPrevOutput=DiscIntNeverNeededParam  ICPrevScaledInput=DiscIntNeverNeededParam
  Discrete-Time Integrator1 : DiscreteIntegrator  InitialCondition=titatm_0  SampleTime=-1  ICPrevOutput=DiscIntNeverNeededParam  ICPrevScaledInput=DiscIntNeverNeededParam
  Discrete-Time Integrator2 : DiscreteIntegrator  SampleTime=-1  ICPrevOutput=DiscIntNeverNeededParam  ICPrevScaledInput=DiscIntNeverNeededParam
  K_wt : Gain  Gain=Lt(2)
  K_θt : Gain  Gain=Lt(1)
  Ki_t : Gain  Gain=Lt(3)
  Sum : Sum  Inputs=|++
  Sum1 : Sum  Inputs=-++
  Sum2 : Sum  Inputs=|++
  Sum3 : Sum  Inputs=|+-
  b_eq : Gain  Gain=bt_eq
  it/rtd : Gain  Gain=it/rtd
  rtd/it : Gain  Gain=rtd/it
  vt_obs : Outport
  wires:
  Sum2/1 -> rtd/it/1, b_eq/1, Discrete-Time Integrator1/1  "wt_obs"
  Discrete-Time Integrator/1 -> Sum2/1
  xtd_enc/1 -> it/rtd/1
  1/J_eq/1 -> Sum/1
  K_θt/1 -> Sum2/2
  Ki_t/1 -> Sum1/3
  Discrete-Time Integrator1/1 -> Sum3/2  "θt_obs"
  Sum/1 -> Discrete-Time Integrator/1  "dot_wt_obs"
  K_wt/1 -> Sum/2
  Ttm_ref/1 -> Sum1/2
  Discrete-Time Integrator2/1 -> Ki_t/1
  Sum3/1 -> Discrete-Time Integrator2/1, K_wt/1, K_θt/1  "e_θt"
  rtd/it/1 -> vt_obs/1
  b_eq/1 -> Sum1/1
  Sum1/1 -> 1/J_eq/1
  it/rtd/1 -> Sum3/1  "θt_enc"

== system modelo_planta_EXPERIMENTAL_prueba/Controlador Izaje/Controlador de Velocidad ==
  m_est : Inport
  vh_ref : Inport  Port=2
  vh_obs : Inport  Port=3
  BRK : Inport  Port=4
  Discrete-Time Integrator : DiscreteIntegrator  IntegratorMethod=Integration: Trapezoidal  ExternalReset=level  SampleTime=-1  ICPrevOutput=DiscIntNeverNeededParam  ICPrevScaledInput=DiscIntNeverNeededParam
  Gain : Gain  Gain=Ki_h
  Gain1 : Gain  Gain=Kp_h
  Gain2 : Gain  Gain=g*rhd/(2*ih)
  Gain3 : Gain  Gain=(2*ih)/rhd
  NOT : Logic  Operator=NOT  IconShape=distinctive  AllPortsSameDT=off  OutDataTypeStr=boolean
  Sum1 : Sum  Inputs=+-
  Sum4 : Sum  Inputs=|++
  Sum5 : Sum  Inputs=|++
  Thm_ref : Outport
  wires:
  Gain1/1 -> Sum4/1
  Sum1/1 -> Gain3/1
  vh_obs/1 -> Sum1/2
  Gain2/1 -> Sum5/2  "Tg_ff"
  Sum5/1 -> Thm_ref/1  "Thm_ref"
  Sum4/1 -> Sum5/1  "T_PID"
  vh_ref/1 -> Sum1/1
  m_est/1 -> Gain2/1
  Discrete-Time Integrator/1 -> Gain/1
  Gain/1 -> Sum4/2
  NOT/1 -> Discrete-Time Integrator/2
  BRK/1 -> NOT/1
  Gain3/1 -> Discrete-Time Integrator/1, Gain1/1  "e_wh"

== system modelo_planta_EXPERIMENTAL_prueba/Controlador Izaje/Modulación de la Referencia ==
  vh_lim : Inport
  seleccion : Inport  Port=2
  vy_cmd : Inport  Port=3
  Constant : Constant  Value=0
  Gain1 : Gain  Gain=-1
  Rate Limiter : RateLimiter  RisingSlewLimit=ah_max  FallingSlewLimit=-ah_max  SampleTimeMode=inherited  InitialCondition=vh_0
  Saturation Dynamic : simulink/Discontinuities/Saturation Dynamic  OutMin=[]  OutMax=[]  OutDataTypeStr=Inherit: Same as second input  OutDataType=fixdt(1, 16)  OutScaling=2^-10  DoSatur=off
  Switch : Switch  Criteria=u2 > Threshold  SaturateOnIntegerOverflow=off  InputSameDT=off
  vh_ref : Outport
  wires:
  Saturation Dynamic/1 -> Rate Limiter/1
  vh_lim/1 -> Gain1/1, Saturation Dynamic/1
  Gain1/1 -> Saturation Dynamic/3
  Rate Limiter/1 -> vh_ref/1
  vy_cmd/1 -> Switch/3
  Switch/1 -> Saturation Dynamic/2  "vh_cmd"
  seleccion/1 -> Switch/2
  Constant/1 -> Switch/1

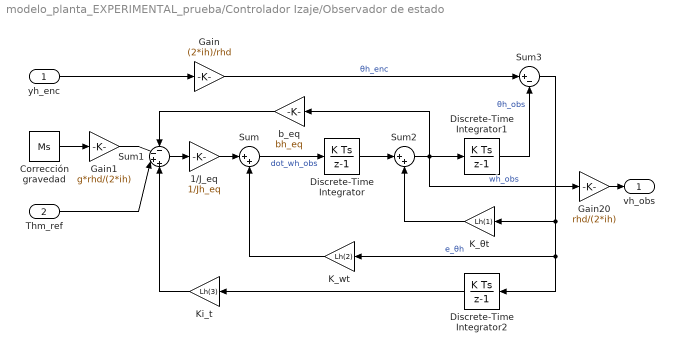
== system modelo_planta_EXPERIMENTAL_prueba/Controlador Izaje/Observador de estado ==
  yh_enc : Inport
  Thm_ref : Inport  Port=2
  1/J_eq : Gain  Gain=1/Jh_eq
  Corrección gravedad : Constant  Value=Ms
  Discrete-Time Integrator : DiscreteIntegrator  InitialCondition=whm_0  SampleTime=-1  ICPrevOutput=DiscIntNeverNeededParam  ICPrevScaledInput=DiscIntNeverNeededParam
  Discrete-Time Integrator1 : DiscreteIntegrator  InitialCondition=titahm_0  SampleTime=-1  ICPrevOutput=DiscIntNeverNeededParam  ICPrevScaledInput=DiscIntNeverNeededParam
  Discrete-Time Integrator2 : DiscreteIntegrator  SampleTime=-1  ICPrevOutput=DiscIntNeverNeededParam  ICPrevScaledInput=DiscIntNeverNeededParam
  Gain : Gain  Gain=(2*ih)/rhd
  Gain1 : Gain  Gain=g*rhd/(2*ih)
  Gain20 : Gain  Gain=rhd/(2*ih)
  K_wt : Gain  Gain=Lh(2)
  K_θt : Gain  Gain=Lh(1)
  Ki_t : Gain  Gain=Lh(3)
  Sum : Sum  Inputs=|++
  Sum1 : Sum  Inputs=--++
  Sum2 : Sum  Inputs=|++
  Sum3 : Sum  Inputs=|+-
  b_eq : Gain  Gain=bh_eq
  vh_obs : Outport
  wires:
  Sum2/1 -> Gain20/1, b_eq/1, Discrete-Time Integrator1/1  "wh_obs"
  Discrete-Time Integrator/1 -> Sum2/1
  yh_enc/1 -> Gain/1
  1/J_eq/1 -> Sum/1
  K_θt/1 -> Sum2/2
  Ki_t/1 -> Sum1/4
  Discrete-Time Integrator1/1 -> Sum3/2  "θh_obs"
  Sum/1 -> Discrete-Time Integrator/1  "dot_wh_obs"
  K_wt/1 -> Sum/2
  Thm_ref/1 -> Sum1/3
  Discrete-Time Integrator2/1 -> Ki_t/1
  Sum3/1 -> Discrete-Time Integrator2/1, K_wt/1, K_θt/1  "e_θh"
  Gain20/1 -> vh_obs/1
  b_eq/1 -> Sum1/1
  Sum1/1 -> 1/J_eq/1
  Gain/1 -> Sum3/1  "θh_enc"
  Corrección gravedad/1 -> Gain1/1
  Gain1/1 -> Sum1/2

== system modelo_planta_EXPERIMENTAL_prueba/Sensores Carro/Encoder Carro ==
  θtm : Inport
  Gain1 : Gain  Gain=rtd/it
  xtd_enc : Outport
  wires:
  θtm/1 -> Gain1/1
  Gain1/1 -> xtd_enc/1

== system modelo_planta_EXPERIMENTAL_prueba/Sensores Carro/Fines de carrera carro (rieles) ==
  xt : Inport
  Compare To Constant : simulink/Logic and Bit Operations/Compare To Constant  relop=>=  const=xt_max  OutDataTypeStr=boolean
  Compare To Constant1 : simulink/Logic and Bit Operations/Compare To Constant  relop=>=  const=xt_max+0.5  OutDataTypeStr=boolean
  Compare To Constant2 : simulink/Logic and Bit Operations/Compare To Constant  relop=<=  const=xt_min  OutDataTypeStr=boolean
  Compare To Constant3 : simulink/Logic and Bit Operations/Compare To Constant  relop=<=  const=xt_min-0.5  OutDataTypeStr=boolean
  FC_derecho : Outport
  FC_izquierdo : Outport  Port=2
  FCE_derecho : Outport  Port=3
  FCE_izquierdo : Outport  Port=4
  wires:
  Compare To Constant2/1 -> FC_izquierdo/1
  xt/1 -> Compare To Constant/1, Compare To Constant1/1, Compare To Constant2/1, Compare To Constant3/1
  Compare To Constant3/1 -> FCE_izquierdo/1
  Compare To Constant1/1 -> FCE_derecho/1
  Compare To Constant/1 -> FC_derecho/1

== system modelo_planta_EXPERIMENTAL_prueba/Sensores Izaje/Encoder Izaje ==
  θhm : Inport
  Gain3 : Gain  Gain=rhd/(2*ih)
  yh_enc : Outport
  wires:
  θhm/1 -> Gain3/1
  Gain3/1 -> yh_enc/1

== system modelo_planta_EXPERIMENTAL_prueba/Sensores Izaje/Fines de carrera izaje (tambor) ==
  y_enc : Inport
  Compare To Constant4 : simulink/Logic and Bit Operations/Compare To Constant  relop=>=  const=yh_max  OutDataTypeStr=boolean
  Compare To Constant5 : simulink/Logic and Bit Operations/Compare To Constant  relop=>=  const=yh_max+0.5  OutDataTypeStr=boolean
  Compare To Constant6 : simulink/Logic and Bit Operations/Compare To Constant  relop=<=  const=yh_min  OutDataTypeStr=boolean
  Compare To Constant7 : simulink/Logic and Bit Operations/Compare To Constant  relop=<=  const=yh_min-0.5  OutDataTypeStr=boolean
  FC_superior : Outport
  FC_inferior : Outport  Port=2
  FCE_superior : Outport  Port=3
  FCE_inferior : Outport  Port=4
  wires:
  Compare To Constant7/1 -> FCE_inferior/1
  y_enc/1 -> Compare To Constant7/1, Compare To Constant6/1, Compare To Constant4/1, Compare To Constant5/1
  Compare To Constant6/1 -> FC_inferior/1
  Compare To Constant5/1 -> FCE_superior/1
  Compare To Constant4/1 -> FC_superior/1

== system modelo_planta_EXPERIMENTAL_prueba/Subsistema Carro/Accionamiento carro ==
  Ftw : Inport
  Ttm : Inport  Port=2
  BRK_t : Inport  Port=3
  Freno Motor : Subsystem
  Ga in1 : Gain  Gain=rtd/it
  Gain : Gain  Gain=1/Jt_eq
  Gain2 : Gain  Gain=rtd/it
  Gain3 : Gain  Gain=bt_eq
  Integrator : Integrator  InitialCondition=wtm_0
  Integrator1 : Integrator  InitialCondition=xtd_0
  Integrator2 : Integrator  InitialCondition=titatm_0
  Sum1 : Sum  Inputs=++--
  θtm : Outport
  xtd : Outport  Port=2
  vtd : Outport  Port=3
  wires:
  Sum1/1 -> Gain/1
  Integrator/1 -> Gain2/1, Freno Motor/2(wtm), Gain3/1, Integrator2/1  "wtm"
  Gain2/1 -> Integrator1/1, vtd/1  "vtd"
  Ttm/1 -> Sum1/1
  Gain/1 -> Integrator/1  "d_wtm"
  BRK_t/1 -> Freno Motor/1(BRK_t)
  Integrator1/1 -> xtd/1
  Ftw/1 -> Ga in1/1
  Ga in1/1 -> Sum1/3
  Freno Motor/1(Ttb) -> Sum1/2
  Gain3/1 -> Sum1/4
  Integrator2/1 -> θtm/1

== system modelo_planta_EXPERIMENTAL_prueba/Subsistema Carro/Dinámica carro ==
  Ftw : Inport
  θl : Inport  Port=2
  Fhw : Inport  Port=3
  Gain : Gain  Gain=2
  Gain1 : Gain  Gain=1/Mt
  Gain2 : Gain  Gain=bt
  Integrator : Integrator  InitialCondition=vt_0
  Integrator1 : Integrator  InitialCondition=xt_0
  Product : Product
  Sin : Trigonometry
  Sum : Sum  Inputs=++-
  xt : Outport
  vt : Outport  Port=2
  at : Outport  Port=3
  wires:
  Gain1/1 -> at/1, Integrator/1  "dot_vt"
  Integrator/1 -> Gain2/1, vt/1, Integrator1/1  "vt"
  Gain2/1 -> Sum/3
  Sum/1 -> Gain1/1
  Integrator1/1 -> xt/1  "xt"
  Fhw/1 -> Gain/1
  Gain/1 -> Product/2
  θl/1 -> Sin/1
  Sin/1 -> Product/1
  Product/1 -> Sum/2  "F_coupling"
  Ftw/1 -> Sum/1

== system modelo_planta_EXPERIMENTAL_prueba/Subsistema Carro/Fuerza cable carro ==
  xtd : Inport
  vtd : Inport  Port=2
  xt : Inport  Port=3
  vt : Inport  Port=4
  Gain : Gain  Gain=Ktw
  Gain1 : Gain  Gain=btw
  Sum : Sum  Inputs=+-
  Sum1 : Sum
  Sum2 : Sum  Inputs=+-
  Ftw : Outport
  wires:
  xtd/1 -> Sum/1
  Gain1/1 -> Sum1/2
  Sum/1 -> Gain/1
  xt/1 -> Sum/2
  Sum2/1 -> Gain1/1
  Gain/1 -> Sum1/1
  vt/1 -> Sum2/2
  Sum1/1 -> Ftw/1  "Ftw"
  vtd/1 -> Sum2/1

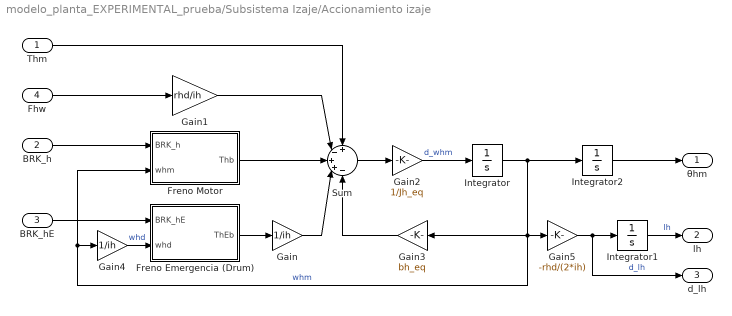
== system modelo_planta_EXPERIMENTAL_prueba/Subsistema Izaje/Accionamiento izaje ==
  Thm : Inport
  BRK_h : Inport  Port=2
  BRK_hE : Inport  Port=3
  Fhw : Inport  Port=4
  Freno Emergencia (Drum) : Subsystem
  Freno Motor : Subsystem
  Gain : Gain  Gain=1/ih
  Gain1 : Gain  Gain=rhd/ih
  Gain2 : Gain  Gain=1/Jh_eq
  Gain3 : Gain  Gain=bh_eq
  Gain4 : Gain  Gain=1/ih
  Gain5 : Gain  Gain=-rhd/(2*ih)
  Integrator : Integrator  InitialCondition=whm_0
  Integrator1 : Integrator  InitialCondition=lh_0
  Integrator2 : Integrator  InitialCondition=titahm_0
  Sum : Sum  Inputs=+-++-
  θhm : Outport
  lh : Outport  Port=2
  d_lh : Outport  Port=3
  wires:
  Gain5/1 -> d_lh/1, Integrator1/1  "d_lh"
  Integrator/1 -> Gain3/1, Freno Motor/2(whm), Gain4/1, Gain5/1, Integrator2/1  "whm"
  Freno Emergencia (Drum)/1(ThEb) -> Gain/1
  Gain3/1 -> Sum/5
  BRK_h/1 -> Freno Motor/1(BRK_h)
  Gain/1 -> Sum/4
  Gain2/1 -> Integrator/1  "d_whm"
  Sum/1 -> Gain2/1
  Gain4/1 -> Freno Emergencia (Drum)/2(whd)  "whd"
  BRK_hE/1 -> Freno Emergencia (Drum)/1(BRK_hE)
  Fhw/1 -> Gain1/1
  Freno Motor/1(Thb) -> Sum/3
  Gain1/1 -> Sum/2
  Integrator1/1 -> lh/1  "lh"
  Integrator2/1 -> θhm/1
  Thm/1 -> Sum/1

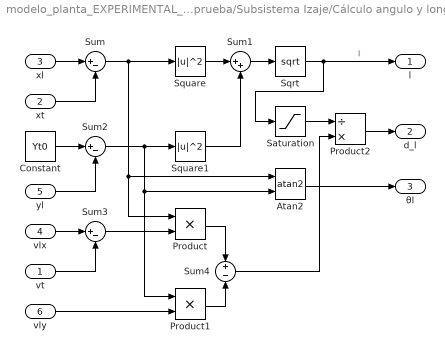
== system modelo_planta_EXPERIMENTAL_prueba/Subsistema Izaje/Cálculo angulo y longitud ==
  vt : Inport
  xt : Inport  Port=2
  xl : Inport  Port=3
  vlx : Inport  Port=4
  yl : Inport  Port=5
  vly : Inport  Port=6
  Atan2 : Trigonometry  Operator=atan2
  Constant : Constant  Value=Yt0
  Product : Product
  Product1 : Product
  Product2 : Product  Inputs=/*
  Saturation : Saturate  UpperLimit=inf  LowerLimit=0.1
  Sqrt : Sqrt
  Square : Math  Operator=magnitude^2
  Square1 : Math  Operator=magnitude^2
  Sum : Sum  Inputs=|+-
  Sum1 : Sum  Inputs=|++
  Sum2 : Sum  Inputs=|+-
  Sum3 : Sum  Inputs=|+-
  Sum4 : Sum  Inputs=+-
  l : Outport
  d_l : Outport  Port=2
  θl : Outport  Port=3
  wires:
  Product2/1 -> d_l/1
  Sqrt/1 -> l/1, Saturation/1  "l"
  Sum1/1 -> Sqrt/1
  Sum2/1 -> Product1/1, Atan2/2, Square1/1
  Sum/1 -> Product/1, Atan2/1, Square/1
  yl/1 -> Sum2/2
  Atan2/1 -> θl/1
  vly/1 -> Product1/2
  xl/1 -> Sum/1
  Constant/1 -> Sum2/1
  Sum3/1 -> Product/2
  Square1/1 -> Sum1/2
  vt/1 -> Sum3/2
  Sum4/1 -> Product2/2
  vlx/1 -> Sum3/1
  xt/1 -> Sum/2
  Square/1 -> Sum1/1
  Product1/1 -> Sum4/2
  Product/1 -> Sum4/1
  Saturation/1 -> Product2/1

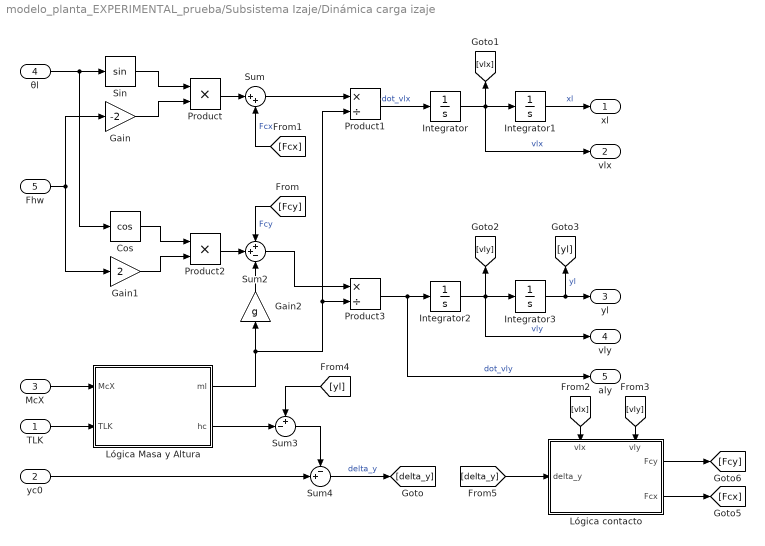
== system modelo_planta_EXPERIMENTAL_prueba/Subsistema Izaje/Dinámica carga izaje ==
  TLK : Inport
  yc0 : Inport  Port=2
  McX : Inport  Port=3
  θl : Inport  Port=4
  Fhw : Inport  Port=5
  Cos : Trigonometry  Operator=cos
  Gain : Gain  Gain=-2
  Gain1 : Gain  Gain=2
  Gain2 : Gain  Gain=g
  Integrator : Integrator  InitialCondition=vlx_0
  Integrator1 : Integrator  InitialCondition=xl_0
  Integrator2 : Integrator  InitialCondition=vly_0
  Integrator3 : Integrator  InitialCondition=yl_0
  Lógica Masa y Altura : Subsystem
  Lógica contacto : Subsystem
      settings: PortSchema="{\"entries\":[{\"content\":{\"sides\":[{\"content\":{\"connectorIds\":[\"In1\"]},\"type\":\"ConnectorPlacement.EquallySpacedRectSide\",\"uuid\":\"20a8b2c4-d5cf-44ce-93ec-929b996a0905\"},{\"content\":{\"connectorIds\":[\"Out1\",\"Out2\"],\"side\":\"RIGHT\"},\"type\":\"ConnectorPlacement.EquallySpacedRectSide\",\"uuid\":\"396e1f2e-cf71-48dc-8d57-a3e2695dfff1\"},{\"content\":{\"connectorIds\":[\"In2\",\"In3\"],\"side\":\"TOP\"},\"type\":\"ConnectorPlacement.EquallySpacedRectSide\",\"uuid\":\"e66c0478-9682-41e1-9b77-d2d789a9c323\"}]},\"type\":\"ConnectorPlacement.EquallySpacedConnector\",\"uuid\":\"193dabd2-f524-433a-b6ef-c1cab585578e\"}],\"packageUris\":[\"http://schema.mathworks.com/mf0/Connector/R2020b\"],\"version\":\"1.0\"}"
  Product : Product
  Product1 : Product  Inputs=*/
  Product2 : Product
  Product3 : Product  Inputs=*/
  Sin : Trigonometry
  Sum : Sum  Inputs=|++
  Sum2 : Sum  Inputs=++-
  Sum3 : Sum  Inputs=+-|
  Sum4 : Sum  Inputs=-+|
  xl : Outport
  vlx : Outport  Port=2
  yl : Outport  Port=3
  vly : Outport  Port=4
  aly : Outport  Port=5
  wires:
  θl/1 -> Sin/1, Cos/1
  Integrator/1 -> vlx/1, Integrator1/1, [vlx]  "vlx"
  Sum3/1 -> Sum4/1
  Sin/1 -> Product/1
  Gain/1 -> Product/2
  [Fcy] -> Sum2/1  "Fcy"
  Integrator2/1 -> vly/1, Integrator3/1, [vly]  "vly"
  Integrator3/1 -> yl/1, [yl]  "yl"
  Fhw/1 -> Gain1/1, Gain/1
  [Fcx] -> Sum/2  "Fcx"
  Product/1 -> Sum/1
  Product1/1 -> Integrator/1  "dot_vlx"
  Gain2/1 -> Sum2/3
  Cos/1 -> Product2/1
  Gain1/1 -> Product2/2
  [yl] -> Sum3/1
  Product2/1 -> Sum2/2
  yc0/1 -> Sum4/2
  Sum2/1 -> Product3/1
  Product3/1 -> aly/1, Integrator2/1  "dot_vly"
  Sum/1 -> Product1/1
  Integrator1/1 -> xl/1  "xl"
  Sum4/1 -> [delta_y]  "delta_y"
  Lógica contacto/1(Fcy) -> [Fcy]
  Lógica contacto/2(Fcx) -> [Fcx]
  Lógica Masa y Altura/1(ml) -> Product1/2, Product3/2, Gain2/1
  McX/1 -> Lógica Masa y Altura/1(McX)
  TLK/1 -> Lógica Masa y Altura/2(TLK)
  Lógica Masa y Altura/2(hc) -> Sum3/2
  [vlx] -> Lógica contacto/2(vlx)
  [vly] -> Lógica contacto/3(vly)
  [delta_y] -> Lógica contacto/1(delta_y)

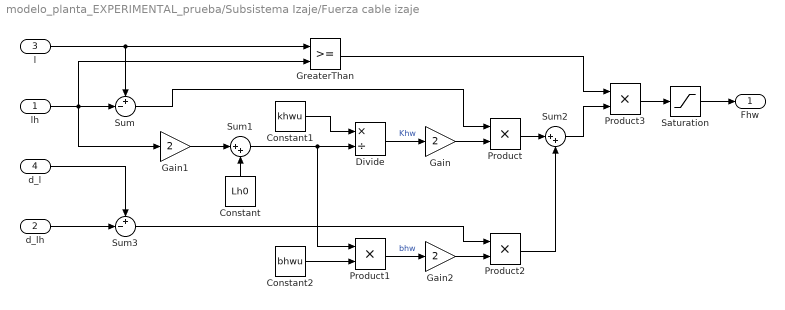
== system modelo_planta_EXPERIMENTAL_prueba/Subsistema Izaje/Fuerza cable izaje ==
  lh : Inport
  d_lh : Inport  Port=2
  l : Inport  Port=3
  d_l : Inport  Port=4
  Constant : Constant  Value=Lh0
  Constant1 : Constant  Value=khwu
  Constant2 : Constant  Value=bhwu
  Divide : Product  Inputs=*/  RndMeth=Zero  SaturateOnIntegerOverflow=on
  Gain : Gain  Gain=2
  Gain1 : Gain  Gain=2
  Gain2 : Gain  Gain=2
  GreaterThan : RelationalOperator  OutDataTypeStr=boolean  RndMeth=Simplest  InputSameDT=off
  Product{,1..3} (4 alike) : Product
  Saturation : Saturate  UpperLimit=inf  LowerLimit=0
  Sum : Sum  Inputs=+-|
  Sum1 : Sum  Inputs=|++
  Sum2 : Sum  Inputs=|++
  Sum3 : Sum  Inputs=+-|
  Fhw : Outport
  wires:
  Constant/1 -> Sum1/2
  Constant2/1 -> Product1/2
  Sum1/1 -> Divide/2, Product1/1
  lh/1 -> Sum/2, GreaterThan/2, Gain1/1
  Product/1 -> Sum2/1
  Gain1/1 -> Sum1/1
  l/1 -> Sum/1, GreaterThan/1
  Product2/1 -> Sum2/2
  Product3/1 -> Saturation/1
  GreaterThan/1 -> Product3/1
  d_lh/1 -> Sum3/2
  Constant1/1 -> Divide/1
  Product1/1 -> Gain2/1  "bhw"
  Sum/1 -> Product/1
  Gain2/1 -> Product2/2
  Divide/1 -> Gain/1  "Khw"
  Sum2/1 -> Product3/2
  Sum3/1 -> Product2/1
  d_l/1 -> Sum3/1
  Gain/1 -> Product/2
  Saturation/1 -> Fhw/1

== system modelo_planta_EXPERIMENTAL_prueba/Subsistema Carro/Accionamiento carro/Freno Motor ==
  BRK_t : Inport
  wtm : Inport  Port=2
  Constant : Constant  Value=0
  Gain3 : Gain  Gain=-Ttb_Max
  Gain4 : Gain  Gain=btb
  Switch : Switch  Criteria=u2 > Threshold  SaturateOnIntegerOverflow=off  InputSameDT=off
  Tanh : Trigonometry  Operator=tanh
  Ttb : Outport
  wires:
  BRK_t/1 -> Switch/2
  Constant/1 -> Switch/1
  wtm/1 -> Gain4/1
  Gain4/1 -> Tanh/1
  Tanh/1 -> Gain3/1
  Gain3/1 -> Switch/3
  Switch/1 -> Ttb/1

== system modelo_planta_EXPERIMENTAL_prueba/Subsistema Izaje/Accionamiento izaje/Freno Emergencia (Drum) ==
  BRK_hE : Inport
  whd : Inport  Port=2
  Constant : Constant  Value=0
  Gain3 : Gain  Gain=-ThEb_Max
  Gain4 : Gain  Gain=bhEb
  Switch : Switch  Criteria=u2 > Threshold  SaturateOnIntegerOverflow=off  InputSameDT=off
  Tanh : Trigonometry  Operator=tanh
  ThEb : Outport
  wires:
  BRK_hE/1 -> Switch/2
  Gain3/1 -> Switch/3
  Constant/1 -> Switch/1
  whd/1 -> Gain4/1
  Gain4/1 -> Tanh/1
  Tanh/1 -> Gain3/1
  Switch/1 -> ThEb/1

== system modelo_planta_EXPERIMENTAL_prueba/Subsistema Izaje/Accionamiento izaje/Freno Motor ==
  BRK_h : Inport
  whm : Inport  Port=2
  Constant : Constant  Value=0
  Gain3 : Gain  Gain=-Thb_Max
  Gain4 : Gain  Gain=bhb
  Switch : Switch  Criteria=u2 > Threshold  SaturateOnIntegerOverflow=off  InputSameDT=off
  Tanh : Trigonometry  Operator=tanh
  Thb : Outport
  wires:
  BRK_h/1 -> Switch/2
  Gain3/1 -> Switch/3
  Constant/1 -> Switch/1
  whm/1 -> Gain4/1
  Gain4/1 -> Tanh/1
  Tanh/1 -> Gain3/1
  Switch/1 -> Thb/1

== system modelo_planta_EXPERIMENTAL_prueba/Subsistema Izaje/Dinámica carga izaje/Lógica Masa y Altura ==
  McX : Inport
  TLK : Inport  Port=2
  Constant : Constant  Value=Ms
  Constant1 : Constant  Value=0
  Constant2 : Constant  Value=Hc
  Rate Limiter : RateLimiter  Commented=through  RisingSlewLimit=Mc_max/0.1  FallingSlewLimit=-Mc_max/0.1  SampleTimeMode=inherited  InitialCondition=Ms
  Sum1 : Sum  Inputs=|++
  Switch : Switch  Criteria=u2 > Threshold  SaturateOnIntegerOverflow=off  InputSameDT=off
  Switch1 : Switch  Criteria=u2 > Threshold  SaturateOnIntegerOverflow=off  InputSameDT=off
  ml : Outport
  hc : Outport  Port=2
  wires:
  Sum1/1 -> Switch/1
  Constant2/1 -> Switch1/1
  TLK/1 -> Switch1/2, Switch/2
  Constant/1 -> Switch/3, Sum1/2
  Constant1/1 -> Switch1/3
  McX/1 -> Sum1/1
  Switch/1 -> Rate Limiter/1
  Rate Limiter/1 -> ml/1
  Switch1/1 -> hc/1

== system modelo_planta_EXPERIMENTAL_prueba/Subsistema Izaje/Dinámica carga izaje/Lógica contacto ==
  delta_y : Inport
  vlx : Inport  Port=2
  vly : Inport  Port=3
  Constant3 : Constant  Value=0
  Constant4 : Constant  Value=0
  Gain3 : Gain  Gain=Kcy
  Gain4 : Gain  Gain=bcy
  Gain5 : Gain  Gain=-bcx
  Saturation : Saturate  UpperLimit=60e5  LowerLimit=0
  Sum5 : Sum  Inputs=-+|
  Switch2 : Switch  SaturateOnIntegerOverflow=off  InputSameDT=off
  Switch3 : Switch  SaturateOnIntegerOverflow=off  InputSameDT=off
  Fcy : Outport
  Fcx : Outport  Port=2
  wires:
  Sum5/1 -> Switch2/1
  vlx/1 -> Gain5/1
  Gain4/1 -> Sum5/1
  vly/1 -> Gain4/1
  Constant4/1 -> Switch3/3
  Gain5/1 -> Switch3/1
  Gain3/1 -> Sum5/2
  delta_y/1 -> Switch3/2, Gain3/1, Switch2/2
  Constant3/1 -> Switch2/3
  Switch2/1 -> Saturation/1  "Fcy"
  Switch3/1 -> Fcx/1  "Fcx"
  Saturation/1 -> Fcy/1
